simulink model "task1"  (R2021b)
settings: Solver=FixedStepAuto  StartTime=0.0  StopTime=5  FixedStep=timeStep  RelTol=1e-3
undefined symbols (not defined in the file): A, B, C
libraries: simulink x1
settings Model: Creator=den  LastModifiedBy=den

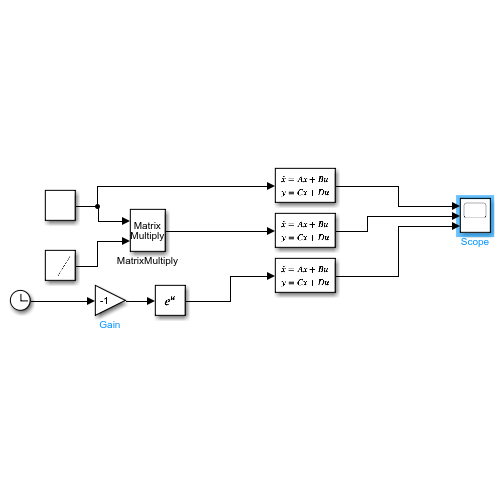
[thumbnail: Simulink's stored preview of the top-level diagram]
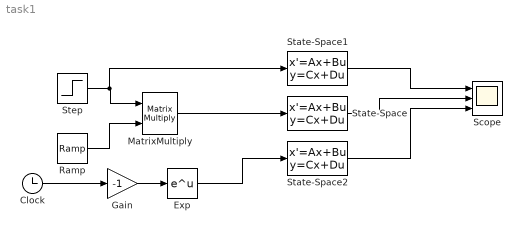
== system task1 ==
  Clock : Clock
  Exp : Math  SaturateOnIntegerOverflow=on
  Gain : Gain  Gain=-1
  MatrixMultiply : Product  Multiplication=Matrix(*)
  Ramp : simulink/Sources/Ramp  slope=-1  start=0  InitialOutput=1
  Scope : Scope  NumInputPorts=3
  State-Space : StateSpace  A=A  B=B  C=C  D=[0; 0]  InitialCondition=0
  State-Space1 : StateSpace  A=A  B=B  C=C  D=[0; 0]  InitialCondition=0
  State-Space2 : StateSpace  A=A  B=B  C=C  D=[0; 0]  InitialCondition=0
  Step : Step  Before=1  After=0  SampleTime=0
  wires:
  Step/1 -> State-Space1/1, MatrixMultiply/1
  Ramp/1 -> MatrixMultiply/2
  MatrixMultiply/1 -> State-Space/1
  Clock/1 -> Gain/1
  Exp/1 -> State-Space2/1
  Gain/1 -> Exp/1
  State-Space2/1 -> Scope/3
  State-Space/1 -> Scope/2
  State-Space1/1 -> Scope/1
